simulink model "gm_hdlcoder_led_blinking_4bit"  (R2016a)
settings: Solver=FixedStepDiscrete  SolverMode=SingleTasking  StartTime=0.0  StopTime=250  RelTol=1e-3
InitFcn:
  | Ts = 1e-3;
libraries: hdlsllib x3, simulink x2
settings Model: Creator=wchen  LastModifiedBy=d57w762
settings DataIOCC: LimitDataPoints=on  SaveFormat=Array  SaveOutput=off  SignalLogging=off  SaveTime=off
settings OptimizationCC: BlockReduction=off  ConditionallyExecuteInputs=off  DefaultParameterBehavior=Inlined  ExpressionDepthLimit=2147483647
settings DebuggingCC: AlgebraicLoopMsg=error  UnderspecifiedInitializationDetection=Classic  MergeDetectMultiDrivingBlocksExec=none  SolverPrmCheckMsg=warning  InheritedTsInSrcMsg=none  SingleTaskRateTransMsg=error  ParameterPrecisionLossMsg=none  StateNameClashWarn=warning
settings HardwareCC: ProdBitPerPointer=32  ProdLargestAtomicFloat=None  ProdIntDivRoundTo=Undefined  ProdEndianess=Unspecified  ProdWordSize=32  ProdHWDeviceType=ASIC/FPGA->ASIC/FPGA  ProdEqTarget=off
settings ModelReferenceCC: PropagateSignalLabelsOutOfModel=off
settings ConfigComp: CovModelRefEnable=Off  CovSFcnEnable=off

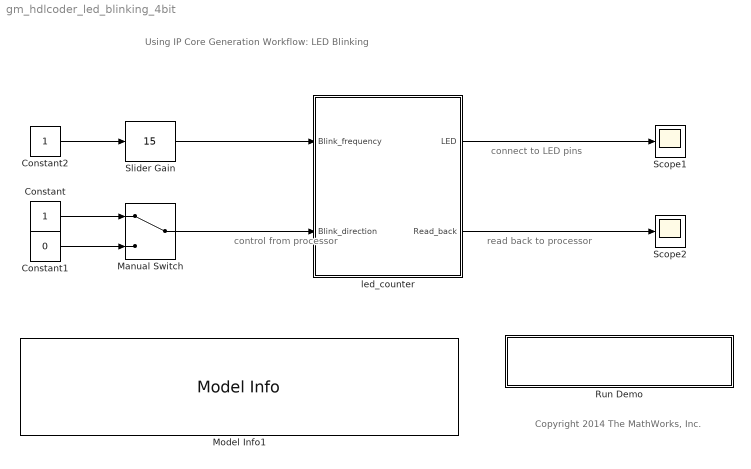
== system gm_hdlcoder_led_blinking_4bit ==
  note: read back to
      | processor
  note: connect to
      | LED pins
  note: control from
      | processor
  note: Using IP Core Generation Workflow: LED Blinking
  note: Copyright 2014 The MathWorks, Inc.
  Constant : Constant  OutDataTypeStr=boolean  SampleTime=Ts
  Constant1 : Constant  Value=0  OutDataTypeStr=boolean  SampleTime=Ts
  Constant2 : Constant  OutDataTypeStr=fixdt(0, 4, 0)  SampleTime=Ts
  Manual Switch : ManualSwitch
  Model Info1 : simulink/Model-Wide Utilities/Model Info  Frame=on  DisplayStringWithTags=|  HorizontalTextAlignment=Left  LeftAlignmentValue=0.02  SourceBlockDiagram=gm_hdlcoder_led_blinking_4bit  TagMaxNumber=20
      | This example shows how to use HDL Workflow Advisor to    
      | generate a custom IP core which blink LEDs on FPGA board.
      |                                                          
      | In MATLAB, type the following:                           
      |   hdladvisor('hdlcoder_led_blinking_4bit/led_counter')
  Run Demo : Subsystem
      settings: OpenFcn=hdladvisor([bdroot, '/led_counter'])
      mask Display: disp('Launch HDL Workflow Advisor')
  Scope1 : Scope
  Scope2 : Scope
  Slider Gain : simulink/Math Operations/Slider Gain  low=0  gain=15  high=15
  led_counter : Subsystem  TreatAsAtomicUnit=on
  wires:
  led_counter/1(LED) -> Scope1/1
  led_counter/2(Read_back) -> Scope2/1
  Slider Gain/1 -> led_counter/1(Blink_frequency)
  Constant2/1 -> Slider Gain/1
  Manual Switch/1 -> led_counter/2(Blink_direction)
  Constant1/1 -> Manual Switch/2
  Constant/1 -> Manual Switch/1

== system gm_hdlcoder_led_blinking_4bit/Run Demo ==

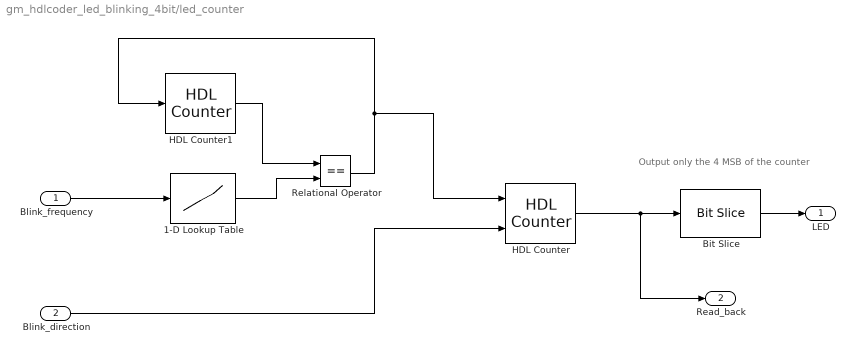
== system gm_hdlcoder_led_blinking_4bit/led_counter ==
  note: Output only the 4 MSB of the counter
  Blink_frequency : Inport  OutDataTypeStr=fixdt(0, 4, 0)
  Blink_direction : Inport  Port=2  OutDataTypeStr=boolean
  1-D Lookup Table : Lookup_n-D  NumberOfTableDimensions=1  BreakpointsForDimension1=[0:15]  IndexSearchMethod=Evenly spaced points  Table=2.^[23:-1:8]  TableDataTypeStr=fixdt(0, 24, 0)  InterpMethod=Flat  DiagnosticForOutOfRangeInput=Error  OutDataTypeStr=fixdt(0, 24, 0)  RndMeth=Simplest  InputSameDT=on
  Bit Slice : hdlsllib/HDL Operations/Bit Slice  lidx=7  ridx=4
  HDL Counter : hdlsllib/HDL Operations/HDL Counter  CountType=Free running  CountInit=0  CountStep=1  CountMax=100  CountFromType=Initial value  CountFrom=0  CountResetPort=off  CountLoadPort=off  CountEnbPort=on  CountDirPort=on  CountDataType=Unsigned  CountWordLen=8  CountFracLen=0  CountSampTime=1
  HDL Counter1 : hdlsllib/HDL Operations/HDL Counter  CountType=Free running  CountInit=0  CountStep=1  CountMax=100  CountFromType=Initial value  CountFrom=0  CountResetPort=on  CountLoadPort=off  CountEnbPort=off  CountDirPort=off  CountDataType=Unsigned  CountWordLen=24  CountFracLen=0  CountSampTime=1
  Relational Operator : RelationalOperator  Operator===  OutDataTypeStr=boolean
  LED : Outport
  Read_back : Outport  Port=2
  wires:
  Bit Slice/1 -> LED/1
  Blink_direction/1 -> HDL Counter/2
  1-D Lookup Table/1 -> Relational Operator/2
  Blink_frequency/1 -> 1-D Lookup Table/1
  Relational Operator/1 -> HDL Counter1/1, HDL Counter/1
  HDL Counter1/1 -> Relational Operator/1
  HDL Counter/1 -> Bit Slice/1, Read_back/1
